simulink library "MinSegLibrary_MinSegNano"  (R2015a)
settings: Solver=ode45  StartTime=0.0  StopTime=10.0  RelTol=1e-3
libraries: arduinolib x4, simulink x2
settings Model: Creator=hurstj  LastModifiedBy=hurstj
settings DebuggingCC: UnderspecifiedInitializationDetection=Classic  MergeDetectMultiDrivingBlocksExec=none  SolverPrmCheckMsg=warning  StateNameClashWarn=warning

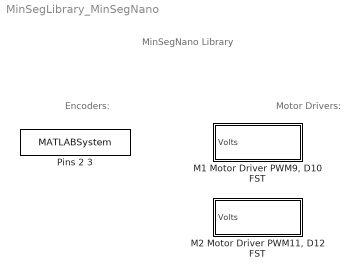
== system MinSegLibrary_MinSegNano ==
  note: Motor Drivers:
  note: Encoders:
  note: MinSegNano Library
  "M1 Motor Driver PWM9, D10 FST" : Subsystem  mask(Motor Driver){Vsupply=3.25}
      mask prompts: Vsupply "Driver Voltage"
      mask help:
      | Use a single PWM and a single Digtial out to control the magnitude and direction of a motor
      |
      | Specify driver supply voltage (3.25 for USB with SN754410)
      mask Display:
      | port_label('input',1,'Volts')
      | text(15,5,['Vsupply=' num2str(Vsupply)])
  "M2 Motor Driver PWM11, D12 FST" : Subsystem  mask(Motor Driver){Vsupply=3.25}
      mask prompts: Vsupply "Driver Voltage"
      mask help:
      | Use a single PWM and a single Digtial out to control the magnitude and direction of a motor
      |
      | Specify driver supply voltage (3.25 for USB with SN754410)
      mask Display:
      | port_label('input',1,'Volts')
      | text(15,5,['Vsupply=' num2str(Vsupply)])
  Pins 2 3 : MATLABSystem  System=Encoder_arduino_uno_nano  Encoder=0  PinA=2  PinB=3
      mask Type: Encoder_arduino_uno_nano
      mask Display:
      | disp('soEncoder');
      | port_label('output',1,'y');

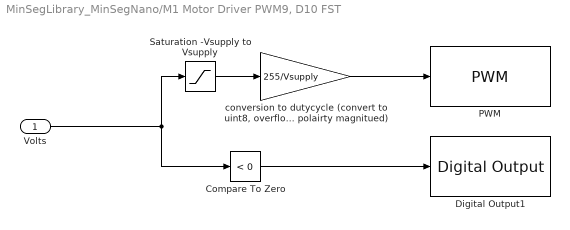
== system MinSegLibrary_MinSegNano/M1 Motor Driver PWM9, D10 FST ==
  Volts : Inport
  Compare To Zero : simulink/Logic and Bit Operations/Compare To Zero  relop=<  OutDataTypeStr=boolean
  Digital Output1 : arduinolib/Digital Output  pinNumber=10  blockPlatform=arduino
  PWM : arduinolib/PWM  pinNumber=9  blockPlatform=arduino
  Saturation -Vsupply to Vsupply : Saturate  UpperLimit=Vsupply  LowerLimit=-Vsupply  OutDataTypeStr=single
  "conversion to dutycycle (convert to uint8, overflow will provide reverse polairty magnitued)" : Gain  Gain=255/Vsupply  OutDataTypeStr=uint8
  wires:
  Volts/1 -> Compare To Zero/1, Saturation -Vsupply to Vsupply/1
  Saturation -Vsupply to Vsupply/1 -> "conversion to dutycycle (convert to uint8, overflow will provide reverse polairty magnitued)"/1
  "conversion to dutycycle (convert to uint8, overflow will provide reverse polairty magnitued)"/1 -> PWM/1
  Compare To Zero/1 -> Digital Output1/1

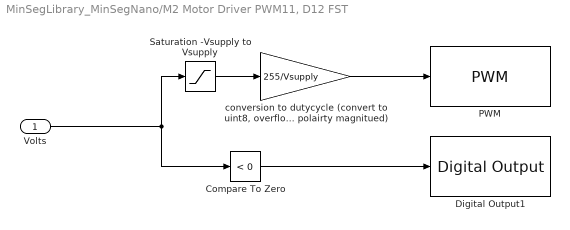
== system MinSegLibrary_MinSegNano/M2 Motor Driver PWM11, D12 FST ==
  Volts : Inport
  Compare To Zero : simulink/Logic and Bit Operations/Compare To Zero  relop=<  OutDataTypeStr=boolean
  Digital Output1 : arduinolib/Digital Output  pinNumber=12  blockPlatform=arduino
  PWM : arduinolib/PWM  pinNumber=11  blockPlatform=arduino
  Saturation -Vsupply to Vsupply : Saturate  UpperLimit=Vsupply  LowerLimit=-Vsupply  OutDataTypeStr=single
  "conversion to dutycycle (convert to uint8, overflow will provide reverse polairty magnitued)" : Gain  Gain=255/Vsupply  OutDataTypeStr=uint8
  wires:
  Compare To Zero/1 -> Digital Output1/1
  "conversion to dutycycle (convert to uint8, overflow will provide reverse polairty magnitued)"/1 -> PWM/1
  Saturation -Vsupply to Vsupply/1 -> "conversion to dutycycle (convert to uint8, overflow will provide reverse polairty magnitued)"/1
  Volts/1 -> Saturation -Vsupply to Vsupply/1, Compare To Zero/1
